simulink model "gm_nrhdlSymbolModulatorModel"  (R2019a)
settings: Solver=FixedStepDiscrete  StartTime=0.0  StopTime=simTime  RelTol=1e-3
libraries: dspsrcs4 x4, ltehdlmod x1
settings Model: Creator=The MathWorks, Inc.  LastModifiedBy=apurvan
settings DataIOCC: SaveOutput=off  SaveTime=off  ReturnWorkspaceOutputs=off
settings OptimizationCC: BlockReduction=off  ConditionallyExecuteInputs=off  DefaultParameterBehavior=Inlined
settings DebuggingCC: AlgebraicLoopMsg=error  InheritedTsInSrcMsg=none  SingleTaskRateTransMsg=error  ArithmeticOperatorsInVariantConditions=warning
settings HardwareCC: ProdBitPerPointer=32  ProdBitPerSizeT=32  ProdBitPerPtrDiffT=32  ProdLargestAtomicFloat=None  ProdIntDivRoundTo=Undefined  ProdEndianess=Unspecified  ProdWordSize=32  ProdHWDeviceType=ASIC/FPGA->ASIC/FPGA  TargetBitPerLong=64  TargetBitPerPointer=64  TargetBitPerSizeT=64  TargetBitPerPtrDiffT=64  TargetLongLongMode=on  TargetIntDivRoundTo=Zero  TargetEndianess=LittleEndian  TargetWordSize=64  TargetHWDeviceType=Custom Processor->MATLAB Host Computer  ProdEqTarget=off

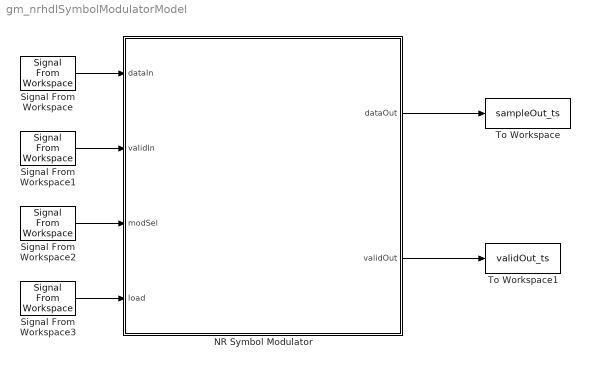
== system gm_nrhdlSymbolModulatorModel ==
  NR Symbol Modulator : Subsystem
  Signal From Workspace : dspsrcs4/Signal From Workspace  X=sampleIn  Ts=sampletime  nsamps=samplesizeIn  OutputAfterFinalValue=Setting to zero  ignoreOrWarnInputAndFrameLengths=off  OutputFrames=off
  Signal From Workspace1 : dspsrcs4/Signal From Workspace  X=validIn  Ts=sampletime  nsamps=samplesizeIn  OutputAfterFinalValue=Setting to zero  ignoreOrWarnInputAndFrameLengths=off  OutputFrames=off
  Signal From Workspace2 : dspsrcs4/Signal From Workspace  X=modSel  Ts=sampletime  nsamps=samplesizeIn  OutputAfterFinalValue=Setting to zero  ignoreOrWarnInputAndFrameLengths=off  OutputFrames=off
  Signal From Workspace3 : dspsrcs4/Signal From Workspace  X=load  Ts=sampletime  nsamps=samplesizeIn  OutputAfterFinalValue=Setting to zero  ignoreOrWarnInputAndFrameLengths=off  OutputFrames=off
  To Workspace : ToWorkspace  VariableName=sampleOut_ts  SaveFormat=Timeseries  SampleTime=-1
  To Workspace1 : ToWorkspace  VariableName=validOut_ts  SaveFormat=Timeseries  SampleTime=-1
  wires:
  Signal From Workspace2/1 -> NR Symbol Modulator/3(modSel)
  Signal From Workspace3/1 -> NR Symbol Modulator/4(load)
  Signal From Workspace1/1 -> NR Symbol Modulator/2(validIn)
  NR Symbol Modulator/1(dataOut) -> To Workspace/1
  Signal From Workspace/1 -> NR Symbol Modulator/1(dataIn)
  NR Symbol Modulator/2(validOut) -> To Workspace1/1

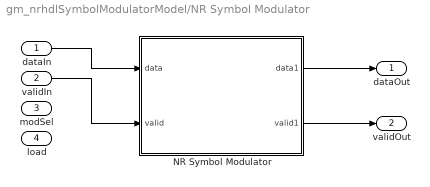
== system gm_nrhdlSymbolModulatorModel/NR Symbol Modulator ==
  dataIn : Inport  OutDataTypeStr=boolean  PortDimensions=1  SampleTime=1
  validIn : Inport  Port=2  OutDataTypeStr=boolean  PortDimensions=1  SampleTime=1
  modSel : Inport  Port=3  OutDataTypeStr=fixdt(0, 3, 0)  PortDimensions=1  SampleTime=1
  load : Inport  Port=4  OutDataTypeStr=boolean  PortDimensions=1  SampleTime=1
  NR Symbol Modulator : Subsystem
  dataOut : Outport
  validOut : Outport  Port=2
  wires:
  dataIn/1 -> NR Symbol Modulator/1(data)
  validIn/1 -> NR Symbol Modulator/2(valid)
  NR Symbol Modulator/1(data1) -> dataOut/1
  NR Symbol Modulator/2(valid1) -> validOut/1

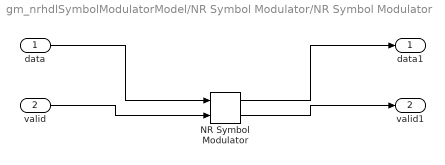
== system gm_nrhdlSymbolModulatorModel/NR Symbol Modulator/NR Symbol Modulator ==
  data : Inport  OutDataTypeStr=boolean  SampleTime=1
  valid : Inport  Port=2  OutDataTypeStr=boolean  SampleTime=1
  NR Symbol Modulator : ltehdlmod/NR Symbol Modulator  ModulationSource=Property  ModulationScheme=QPSK  SimulateUsing=Code generation  OutputDataType=Custom  WordLength=outWordLength
      settings: SourceProductName=LTE HDL Toolbox  SourceProductBaseCode=LH
  data1 : Outport
  valid1 : Outport  Port=2
  wires:
  data/1 -> NR Symbol Modulator/1
  valid/1 -> NR Symbol Modulator/2
  NR Symbol Modulator/1 -> data1/1
  NR Symbol Modulator/2 -> valid1/1
